simulink model "ISO2631Simulation"  (Simulink 7.6)
settings: Solver=FixedStepDiscrete  StartTime=0.0  StopTime=1  RelTol=1e-3
libraries: simulink x1
settings Model: Creator=Kristian  LastModifiedBy=Kristian
settings OptimizationCC: UseSpecifiedMinMax=on  EnhancedBackFolding=on  ZeroExternalMemoryAtStartup=off  ZeroInternalMemoryAtStartup=off  EfficientFloat2IntCast=on  OptimizeModelRefInitCode=on  LifeSpan=1
settings HardwareCC: ProdBitPerChar=16  ProdBitPerInt=16  ProdBitPerPointer=16  ProdLargestAtomicInteger=Integer  ProdIntDivRoundTo=Zero  ProdEndianess=LittleEndian  ProdWordSize=16  ProdHWDeviceType=Texas Instruments->C2000
settings RTWCC: SystemTargetFile=autosar.tlc  GenCodeOnly=on  TemplateMakefile=ert_default_tmf  Description=AUTOSAR  GenerateReport=on  ProcessScript=autosar_make_rtw_hook  IncludeHyperlinkInReport=on  LaunchReport=on  GenerateTraceInfo=on  GenerateTraceReport=on  GenerateTraceReportSl=on  GenerateTraceReportSf=on  GenerateTraceReportEml=on  RTWCompilerOptimization=On
settings CodeAppCC: IgnoreCustomStorageClasses=off
settings STFCustomTargetCC: ParMdlRefBuildCompliant=on  CompOptLevelCompliant=on  IncludeMdlTerminateFcn=off  CombineOutputUpdateFcns=on  CombineSignalStateStructs=on  SuppressErrorStatus=on  ERTFirstTimeCompliant=on  ERTCustomFileBanners=on  SupportNonFinite=off  SupportComplex=off  SupportContinuousTime=off  SupportNonInlinedSFcns=off  AutosarCompliant=on  SystemTargetFile=autosar.tlc
settings ERTTargetCC: MultiwordLength=2048  IncludeMdlTerminateFcn=off  CombineSignalStateStructs=on  SuppressErrorStatus=on  SupportNonFinite=off  SupportComplex=off  ModelStepFunctionPrototypeControlCompliant=off  CPPClassGenCompliant=off  AutosarCompliant=on  ExtModeMexFile=noextcomm  InlinedParameterPlacement=NonHierarchical  ERTCustomFileTemplate=example_file_process.tlc
settings CustomProperty: DataType=RTWOptions_EnumType__toolbox_rtw_targets_AUTOSAR_AUTOSAR_autosar_1_1AutosarSchemaVersion  Value=3.1
settings EnumStrPairs: String=2.0

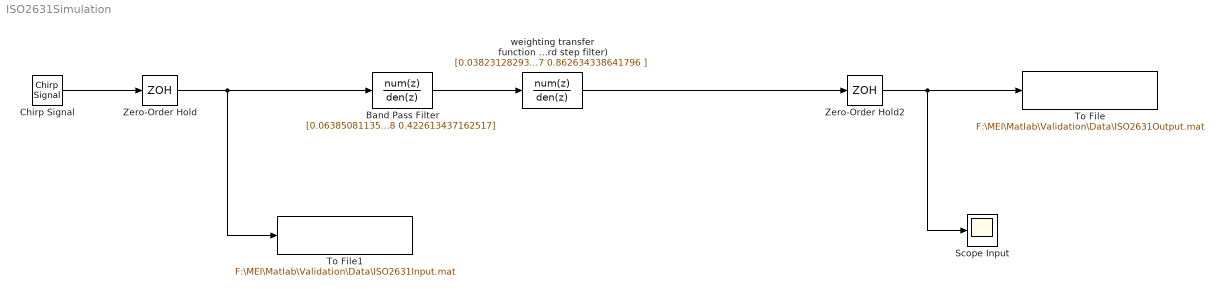
== system ISO2631Simulation ==
  Band Pass Filter : DiscreteFilter  Numerator=|  Denominator=[1.0 -3.16470636644551 3.75293919582273 -2.01084465327318 0.422613437162517]  SampleTime=1/1000
      | [0.0638508113542868 1.33226762955019E-15 -0.127701622708578 4.2188474935756E-15 0.0638508113542855
      | ]
  Chirp Signal : simulink/Sources/Chirp Signal  SystemSampleTime=-1  f1=0.1  T=1  f2=400  VectorParams1D=off
  Scope Input : Scope
  To File : ToFile  Filename=F:\MEI\Matlab\Validation\Data\ISO2631Output.mat  MatrixName=ISO2631Output
  To File1 : ToFile  Filename=F:\MEI\Matlab\Validation\Data\ISO2631Input.mat  MatrixName=ISO2631Input
  Zero-Order Hold : ZeroOrderHold  SampleTime=1/1000
  Zero-Order Hold2 : ZeroOrderHold  SampleTime=1/1000
  weighting transfer function (Acceleration-velocity transition + Upward step filter) : DiscreteFilter  Numerator=|  Denominator=|  SampleTime=1/1000
      Numerator=|
      | [0.0382312829345277 -0.0729444373075823 -0.0034621921267961 0.0729450727468253 -0.0347684553684901
      | ]
      Denominator=|
      | [1.0 -3.85371908982878 5.57025894073329 -3.57917165034607 0.862634338641796
      | ]
  wires:
  Band Pass Filter/1 -> weighting transfer function (Acceleration-velocity transition + Upward step filter)/1
  weighting transfer function (Acceleration-velocity transition + Upward step filter)/1 -> Zero-Order Hold2/1
  Chirp Signal/1 -> Zero-Order Hold/1
  Zero-Order Hold/1 -> Band Pass Filter/1, To File1/1
  Zero-Order Hold2/1 -> To File/1, Scope Input/1
